simulink library "Latency_lib"  (Simulink 7.2)
settings: Solver=ode45  SolverMode=SingleTasking  StartTime=0.0  StopTime=10.0  RelTol=1e-3
undefined symbols (not defined in the file or in its folder): Timestep
libraries: simulink x2
settings Model: Creator=cbuttril  LastModifiedBy=amurch

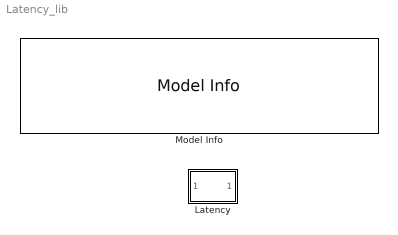
== system Latency_lib ==
  Latency : Subsystem  mask(Latency ){Latency=.02}
      mask prompts: Latency "Desired latency (sec)"
      mask help:
      | Add latency (time delay) to a signal. This blocks implements a
      | discrete delay, based on the simulation's sample-time ('Timestep').
      | Only integer multiples of the base sample time can be used.
      | All input signals should be in a vector, not a bus.
      mask Display: fprintf([num2str(Latency*1000) '\n msec'])
  Model Info : simulink/Model-Wide Utilities/Model Info  SystemSampleTime=-1  InitialBlockCM=None  BlockCM=None  Frame=on  DisplayStringWithTags=|  HorizontalTextAlignment=Center  LeftAlignmentValue=0.5  SourceBlockDiagram=Latency_lib  TagMaxNumber=20
      | Developed using Matlab Release 2007a
      | 
      | SVN:%<ModelVersion>
      | Last modifed by %<LastModifiedBy> on %<LastModificationDate>

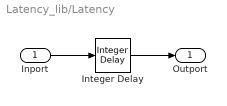
== system Latency_lib/Latency ==
  Inport : Inport  OutDataType=sfix(16)  OutScaling=2^0
  Integer Delay : simulink/Discrete/Integer Delay  vinit=0.0  samptime=Timestep  NumDelays=round(Latency/Timestep)
  Outport : Outport  OutDataType=sfix(16)  OutScaling=2^0
  wires:
  Inport/1 -> Integer Delay/1
  Integer Delay/1 -> Outport/1
